simulink model "Wireless_Charging_Old_V1"  (R2022b)
settings: Solver=VariableStepAuto  StartTime=0.0  StopTime=5  RelTol=1e-3
libraries: spsVoltageMeasurementLib x16, spsSeriesRLCBranchLib x12, spsDiodeLib x11, spsIGBTDiodeLib x9, spsCurrentMeasurementLib x7, spsMosfetLib x2, spsACVoltageSourceLib x1, spsPWMGeneratorDCDCLib x1, spsPWMGenerator2LevelLib x1, spsGroundLib x1, spsMutualInductanceLib x1, spspowerguiLib x1
settings Model: Creator=hp  LastModifiedBy=Aryan Aggarwal
settings OptimizationCC: ReuseModelBlockBuffer=on

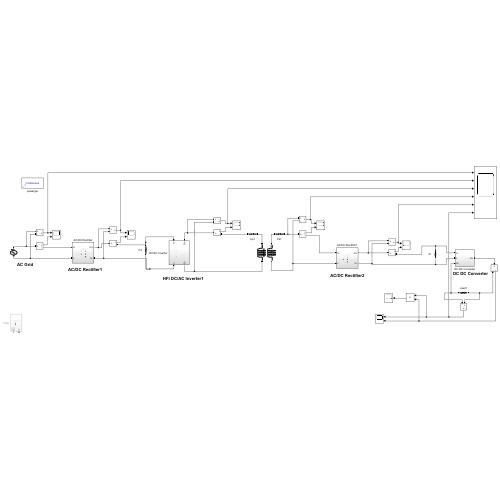
[thumbnail: Simulink's stored preview of the top-level diagram]
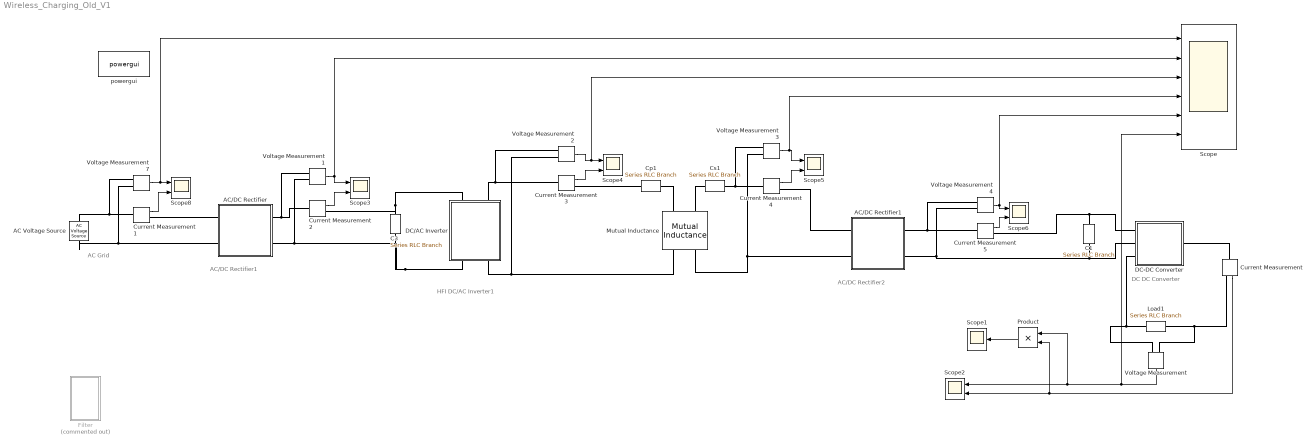
== system Wireless_Charging_Old_V1 ==
  note: AC/DC Rectifier1
  note: AC Grid
  note: HFI DC/AC Inverter1
  note: AC/DC Rectifier2
  note: DC DC Converter
  AC Voltage Source : spsACVoltageSourceLib/AC Voltage Source  Amplitude=230  Phase=0  Frequency=50  SampleTime=0  Measurements=None  BusType=swing  Pref=10e3  Qref=0  Qmin=-inf  Qmax=+inf
  AC/DC Rectifier : Subsystem
  AC/DC Rectifier1 : Subsystem
  C1 : spsSeriesRLCBranchLib/Series RLC Branch  LConnTagsString=__new0  RConnTagsString=__new0  BranchType=C  Resistance=1  Inductance=1e-3  SetiL0=off  InitialCurrent=0  Capacitance=1  Setx0=off  InitialVoltage=0  Measurements=None
  C3 : spsSeriesRLCBranchLib/Series RLC Branch  LConnTagsString=__new0  RConnTagsString=__new0  BranchType=C  Resistance=1  Inductance=1e-3  SetiL0=off  InitialCurrent=0  Capacitance=1  Setx0=off  InitialVoltage=0  Measurements=None
  Cp1 : spsSeriesRLCBranchLib/Series RLC Branch  LConnTagsString=__new0  RConnTagsString=__new0  BranchType=C  Resistance=1  Inductance=1e-3  SetiL0=off  InitialCurrent=0  Capacitance=4.67e-03  Setx0=off  InitialVoltage=0  Measurements=None
  Cs1 : spsSeriesRLCBranchLib/Series RLC Branch  LConnTagsString=__new0  RConnTagsString=__new0  BranchType=C  Resistance=1  Inductance=1e-3  SetiL0=off  InitialCurrent=0  Capacitance=4.67e-03  Setx0=off  InitialVoltage=0  Measurements=None
  Current Measurement{,1..5} (6 alike) : spsCurrentMeasurementLib/Current Measurement  PhasorSimulation=off  OutputType=Complex  PSBequivalent=0
  DC-DC Converter : Subsystem
  DC/AC Inverter : Subsystem
  Filter : Subsystem  Commented=on
  Load1 : spsSeriesRLCBranchLib/Series RLC Branch  LConnTagsString=__new0  RConnTagsString=__new0  BranchType=R  Resistance=100  Inductance=1e-3  SetiL0=off  InitialCurrent=0  Capacitance=1000e-6  Setx0=off  InitialVoltage=0  Measurements=None
  Mutual Inductance : spsMutualInductanceLib/Mutual Inductance  LConnTagsString=a|b  RConnTagsString=A|B  TypeOfMutual=Two or three windings with equal mutual terms  NumberOfWindings=3  SelfImpedance1=[1.1 30e-03]  SelfImpedance2=[ 1.1 30e-03]  ThreeWindings=off  SelfImpedance3=[ 1.1 1.1e-03]  MutualImpedance=[1.0 29e-03]  InductanceMatrix="[1.0 0.9  0.9 ;  0.9 1.0  0.9;  0.9 0.9 1.0 ] * 1e-3"  ResistanceMatrix="[1.0 0.9  0.9 ;  0.9 1.0  0.9;  0.9 0.9 1.0 ]"  Measurements=None
      settings: LibrarySourceBlock=sps_lib/Passives/Mutual Inductance
  Product : Product
  Scope : Scope  NumInputPorts=6
  Scope1 : Scope
  Scope{2..6,8} (6 alike) : Scope  NumInputPorts=2
  Voltage Measurement{,1..4,7} (6 alike) : spsVoltageMeasurementLib/Voltage Measurement  PhasorSimulation=off  OutputType=Complex  PSBequivalent=0
  powergui : spspowerguiLib/powergui  Priority=1  SimulationMode=Continuous  SampleTime=50e-6  frequency=60  Iterations=50  frequencyindice=0  Pbase=100e6  ErrMax=1e-4  UnitsV=kV  UnitsW=MW  buscounter=0  FunctionMessages=off  echomessages=off  EnableUseOfTLC=off  CurrentSourceSwitches=off  DisableSnubberDevices=off  DisableRonSwitches=off  DisableVfSwitches=off  DisplayEquations=off  AutomaticDiscreteSolvers=off  SolverType=Tustin/Backward Euler (TBE)  Interpol=off  ExternalGateDelay=off  methode=off  Ts=100  x0status=blocks  SPID=on  SwTol=0  HookPort=off  NonlinearTolerance=1e-4  nMaxIteration=100  ContinueOnMaxIteration=off  RestoreLinks=warning  ResistiveCurrentMeasurement=off  Frange=[0:2:500]  Ylog=off  Xlog=on  ShowGrid=off  save=off  variable=ZData  structure=0  ZoomFFT=off  StartTime=0.0  cycles=1  DisplayStyle=1  fundamental=60  FreqAxis=off  MaxFrequency=1000  frequencyindicesteady=1  RmsSteady=1  display=off
  wires:
  Product/1 -> Scope1/1
  Voltage Measurement7/1 -> Scope/1, Scope8/1
  Current Measurement1/1 -> Scope8/2
  Voltage Measurement1/1 -> Scope3/1, Scope/2
  Current Measurement2/1 -> Scope3/2
  Voltage Measurement2/1 -> Scope/3, Scope4/1
  Current Measurement3/1 -> Scope4/2
  Voltage Measurement3/1 -> Scope/4, Scope5/1
  Current Measurement4/1 -> Scope5/2
  Voltage Measurement4/1 -> Scope6/1, Scope/5
  Current Measurement5/1 -> Scope6/2
  Voltage Measurement/1 -> Scope2/1, Product/1, Scope/6
  Current Measurement/1 -> Scope2/2, Product/2
  connections:
  Current Measurement/LConn1 -- DC-DC Converter/RConn1
  C1/RConn1 -- DC-DC Converter/LConn2 -- Voltage Measurement4/LConn2 -- AC/DC Rectifier1/LConn2
  Voltage Measurement3/LConn2 -- Mutual Inductance/RConn2 -- AC/DC Rectifier1/RConn2
  DC-DC Converter/LConn3 -- Load1/RConn1 -- Voltage Measurement/LConn2
  Current Measurement5/RConn1 -- C1/LConn1 -- DC-DC Converter/LConn1
  DC/AC Inverter/RConn2 -- Voltage Measurement2/LConn2 -- Mutual Inductance/RConn1
  Voltage Measurement/LConn1 -- Load1/LConn1 -- Current Measurement/RConn1
  Cp1/RConn1 -- Mutual Inductance/LConn1
  AC Voltage Source/LConn1 -- Voltage Measurement7/LConn2 -- AC/DC Rectifier/RConn2
  Cs1/LConn1 -- Mutual Inductance/LConn2
  Current Measurement1/RConn1 -- AC/DC Rectifier/RConn1
  Current Measurement1/LConn1 -- Voltage Measurement7/LConn1 -- AC Voltage Source/RConn1
  C3/LConn1 -- Current Measurement2/RConn1 -- DC/AC Inverter/LConn1
  C3/RConn1 -- Voltage Measurement1/LConn2 -- AC/DC Rectifier/LConn2 -- DC/AC Inverter/RConn1
  Current Measurement2/LConn1 -- Voltage Measurement1/LConn1 -- AC/DC Rectifier/LConn1
  Current Measurement3/LConn1 -- Voltage Measurement2/LConn1 -- DC/AC Inverter/LConn2
  Current Measurement3/RConn1 -- Cp1/LConn1
  Current Measurement4/LConn1 -- Voltage Measurement3/LConn1 -- Cs1/RConn1
  Current Measurement4/RConn1 -- AC/DC Rectifier1/RConn1
  Current Measurement5/LConn1 -- Voltage Measurement4/LConn1 -- AC/DC Rectifier1/LConn1

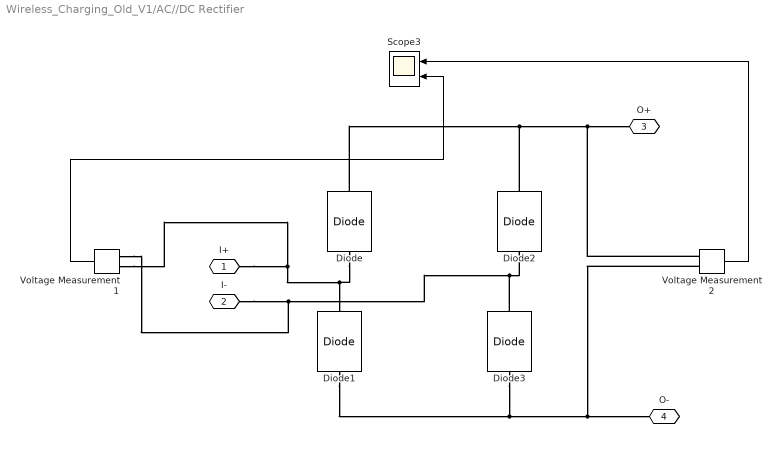
== system Wireless_Charging_Old_V1/AC//DC Rectifier ==
  Diode{,1..3} (4 alike) : spsDiodeLib/Diode  Ron=0.001  Lon=0  Vf=0.8  IC=0  UseSnubber=0  Rs=500  Cs=250e-9  Measurements=off
  Scope3 : Scope  NumInputPorts=2
  Voltage Measurement1 : spsVoltageMeasurementLib/Voltage Measurement  PhasorSimulation=off  OutputType=Complex  PSBequivalent=0
  Voltage Measurement2 : spsVoltageMeasurementLib/Voltage Measurement  PhasorSimulation=off  OutputType=Complex  PSBequivalent=0
  I+ : PMIOPort  Side=Right
  I- : PMIOPort  Port=2  Side=Right
  O+ : PMIOPort  Port=3  Side=Left
  O- : PMIOPort  Port=4  Side=Left
  wires:
  Voltage Measurement2/1 -> Scope3/1
  Voltage Measurement1/1 -> Scope3/2
  connections:
  Diode3/RConn1 -- Voltage Measurement1/LConn2 -- I-/RConn1 -- Diode2/LConn1
  Diode/LConn1 -- Voltage Measurement1/LConn1 -- I+/RConn1 -- Diode1/RConn1
  Diode/RConn1 -- Voltage Measurement2/LConn1 -- O+/RConn1 -- Diode2/RConn1
  Diode1/LConn1 -- Diode3/LConn1 -- Voltage Measurement2/LConn2 -- O-/RConn1

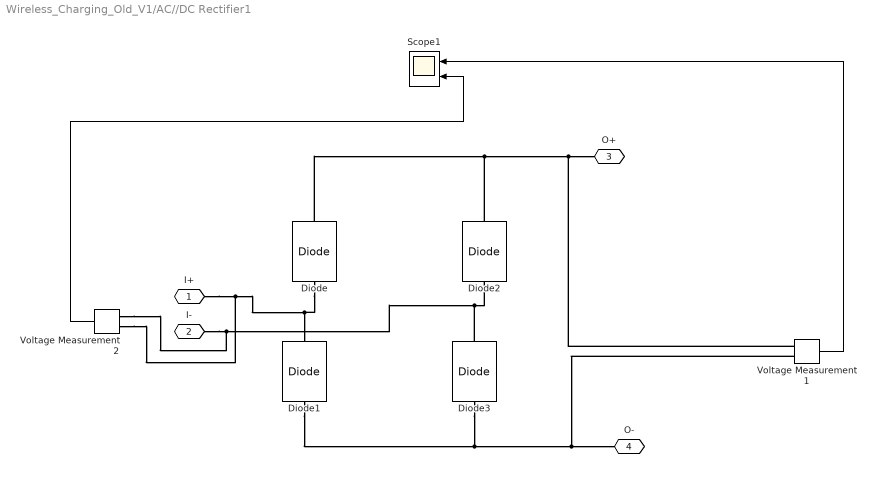
== system Wireless_Charging_Old_V1/AC//DC Rectifier1 ==
  Diode{,1..3} (4 alike) : spsDiodeLib/Diode  Ron=0.001  Lon=0  Vf=0.8  IC=0  UseSnubber=0  Rs=500  Cs=250e-9  Measurements=off
  Scope1 : Scope  NumInputPorts=2
  Voltage Measurement1 : spsVoltageMeasurementLib/Voltage Measurement  PhasorSimulation=off  OutputType=Complex  PSBequivalent=0
  Voltage Measurement2 : spsVoltageMeasurementLib/Voltage Measurement  PhasorSimulation=off  OutputType=Complex  PSBequivalent=0
  I+ : PMIOPort  Side=Right
  I- : PMIOPort  Port=2  Side=Right
  O+ : PMIOPort  Port=3  Side=Left
  O- : PMIOPort  Port=4  Side=Left
  wires:
  Voltage Measurement1/1 -> Scope1/1
  Voltage Measurement2/1 -> Scope1/2
  connections:
  Diode3/RConn1 -- Voltage Measurement2/LConn2 -- I-/RConn1 -- Diode2/LConn1
  Diode/LConn1 -- Voltage Measurement2/LConn1 -- I+/RConn1 -- Diode1/RConn1
  Diode/RConn1 -- Diode2/RConn1 -- Voltage Measurement1/LConn1 -- O+/RConn1
  Diode1/LConn1 -- Diode3/LConn1 -- Voltage Measurement1/LConn2 -- O-/RConn1

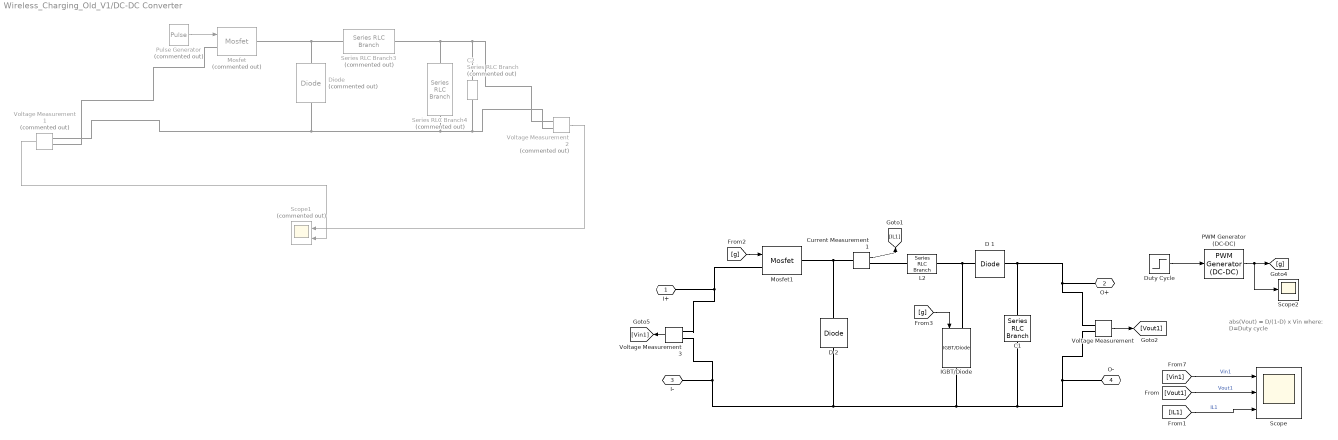
== system Wireless_Charging_Old_V1/DC-DC Converter ==
  note: abs(Vout) = D/(1-D) x Vin
      | where: D=Duty cycle
  C1 : spsSeriesRLCBranchLib/Series RLC Branch  LConnTagsString=__new0  RConnTagsString=__new0  BranchType=C  Resistance=1e-4  Inductance=200e-6  SetiL0=off  InitialCurrent=0  Capacitance=2000e-6  Setx0=on  InitialVoltage=7.5  Measurements=None
  C2 : spsSeriesRLCBranchLib/Series RLC Branch  Commented=on  LConnTagsString=__new0  RConnTagsString=__new0  BranchType=C  Resistance=1  Inductance=1e-3  SetiL0=off  InitialCurrent=0  Capacitance=1  Setx0=off  InitialVoltage=0  Measurements=None
  Current Measurement1 : spsCurrentMeasurementLib/Current Measurement  PhasorSimulation=off  OutputType=Complex  PSBequivalent=0
  D 1 : spsDiodeLib/Diode  Ron=1e-3  Lon=0  Vf=0  IC=0  UseSnubber=off  Rs=inf  Cs=inf  Measurements=off
  D 2 : spsDiodeLib/Diode  Ron=1e-3  Lon=0  Vf=0  IC=0  UseSnubber=off  Rs=inf  Cs=inf  Measurements=off
  Diode : spsDiodeLib/Diode  Commented=on  Ron=0.001  Lon=0  Vf=0.8  IC=0  UseSnubber=0  Rs=500  Cs=250e-9  Measurements=off
  Duty Cycle : Step  Time=0.015  Before=0.456  After=0.602  SampleTime=0
  IGBT/Diode : spsIGBTDiodeLib/IGBT//Diode  Ron=1e-3  Rs=1e5  Cs=inf  Measurements=off
  L2 : spsSeriesRLCBranchLib/Series RLC Branch  LConnTagsString=__new0  RConnTagsString=__new0  BranchType=L  Resistance=1e-4  Inductance=750e-6  SetiL0=on  InitialCurrent=14  Capacitance=30e-6  Setx0=off  InitialVoltage=150  Measurements=None
  Mosfet : spsMosfetLib/Mosfet  Commented=on  Ron=0.1  Lon=0  Rd=0.01  Vfd=0  IC=0  Rs=1e5  Cs=inf  Measurements=off
  Mosfet1 : spsMosfetLib/Mosfet  Ron=1e-3  Lon=0  Rd=1e-3  Vfd=0  IC=0  Rs=1e6  Cs=inf  Measurements=off
  PWM Generator (DC-DC) : spsPWMGeneratorDCDCLib/PWM Generator (DC-DC)  Fsw=10e3  Ts=0
  Pulse Generator : DiscretePulseGenerator  Commented=on  PulseType=Time based  Period=1/100  PulseWidth=80
  Scope : Scope  NumInputPorts=3
  Scope1 : Scope  Commented=on  NumInputPorts=2
  Scope2 : Scope
  Series RLC Branch3 : spsSeriesRLCBranchLib/Series RLC Branch  Commented=on  LConnTagsString=__new0  RConnTagsString=__new0  BranchType=L  Resistance=1  Inductance=50e-3  SetiL0=off  InitialCurrent=0  Capacitance=1e-6  Setx0=off  InitialVoltage=0  Measurements=None
  Series RLC Branch4 : spsSeriesRLCBranchLib/Series RLC Branch  Commented=on  LConnTagsString=__new0  RConnTagsString=__new0  BranchType=C  Resistance=1  Inductance=1e-3  SetiL0=off  InitialCurrent=0  Capacitance=100e-6  Setx0=off  InitialVoltage=0  Measurements=None
  Voltage Measurement : spsVoltageMeasurementLib/Voltage Measurement  PhasorSimulation=off  OutputType=Complex  PSBequivalent=0
  Voltage Measurement1 : spsVoltageMeasurementLib/Voltage Measurement  Commented=on  PhasorSimulation=off  OutputType=Complex  PSBequivalent=0
  Voltage Measurement2 : spsVoltageMeasurementLib/Voltage Measurement  Commented=on  PhasorSimulation=off  OutputType=Complex  PSBequivalent=0
  Voltage Measurement3 : spsVoltageMeasurementLib/Voltage Measurement  PhasorSimulation=off  OutputType=Complex  PSBequivalent=0
  I+ : PMIOPort  Side=Left
  O+ : PMIOPort  Port=2  Side=Right
  I- : PMIOPort  Port=3  Side=Left
  O- : PMIOPort  Port=4  Side=Left
  wires:
  Pulse Generator/1 -> Mosfet/1
  Voltage Measurement1/1 -> Scope1/2
  Voltage Measurement2/1 -> Scope1/1
  Current Measurement1/1 -> [IL1]
  [g] -> IGBT/Diode/1
  Voltage Measurement/1 -> [Vout1]
  [g] -> Mosfet1/1
  Voltage Measurement3/1 -> [Vin1]
  Duty Cycle/1 -> PWM Generator (DC-DC)/1
  PWM Generator (DC-DC)/1 -> Scope2/1, [g]
  [IL1] -> Scope/3  "IL1"
  [Vout1] -> Scope/2  "Vout1"
  [Vin1] -> Scope/1  "Vin1"
  connections:
  Series RLC Branch3/LConn1 -- Mosfet/RConn1 -- Diode/RConn1
  Series RLC Branch4/LConn1 -- Series RLC Branch3/RConn1 -- C2/RConn1 -- Voltage Measurement2/LConn1
  Voltage Measurement2/LConn2 -- Series RLC Branch4/RConn1 -- Voltage Measurement1/LConn2 -- Diode/LConn1 -- C2/LConn1
  Voltage Measurement1/LConn1 -- Mosfet/LConn1
  IGBT/Diode/LConn1 -- D 1/LConn1 -- L2/RConn1
  Voltage Measurement/LConn2 -- C1/RConn1 -- IGBT/Diode/RConn1 -- D 2/LConn1 -- Voltage Measurement3/LConn2 -- I-/RConn1 -- O-/RConn1
  Voltage Measurement/LConn1 -- C1/LConn1 -- D 1/RConn1 -- O+/RConn1
  I+/RConn1 -- Mosfet1/LConn1 -- Voltage Measurement3/LConn1
  Current Measurement1/LConn1 -- Mosfet1/RConn1 -- D 2/RConn1
  L2/LConn1 -- Current Measurement1/RConn1

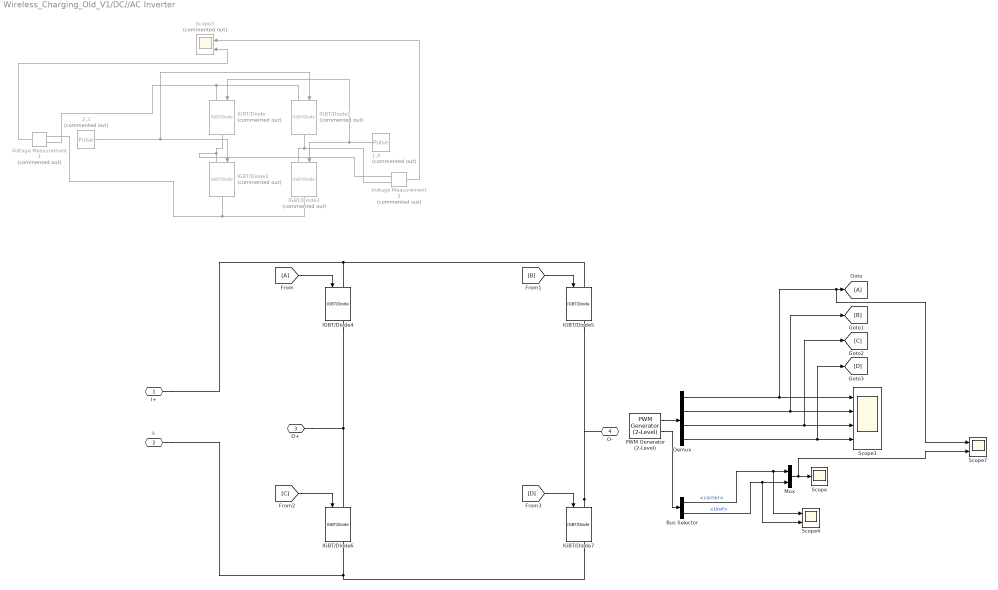
== system Wireless_Charging_Old_V1/DC//AC Inverter ==
  1,4 : DiscretePulseGenerator  Commented=on  PulseType=Time based  Amplitude=15  Period=1/50  PulseWidth=50  PhaseDelay=1/100
  2,3 : DiscretePulseGenerator  Commented=on  PulseType=Time based  Amplitude=15  Period=1/50  PulseWidth=50
  Bus Selector : BusSelector  OutputSignals=carrier,Uref
  Demux : Demux
  From : From
  Goto : Goto
  IGBT/Diode{,1..3} (4 alike) : spsIGBTDiodeLib/IGBT//Diode  Commented=on  Ron=1e-3  Rs=1e5  Cs=inf  Measurements=off
  IGBT/Diode{4..7} (4 alike) : spsIGBTDiodeLib/IGBT//Diode  Ron=1e-3  Rs=1e5  Cs=inf  Measurements=on
  Mux : Mux  Inputs=2
  PWM Generator (2-Level) : spsPWMGenerator2LevelLib/PWM Generator (2-Level)  ModulatorType=Single-phase full-bridge - Bipolar modulation (4 pulses)  ModulatorMode=Unsynchronized  Fc=20000  Pc=0  nF=27  MinMax="[ -1  1 ]"  SamplingTechnique=Asymmetrical regular (double edge)  ModulatingSignals=on  m=0.75  Freq=60  Phase=0  Ts=0  ShowCarrierOutport=on
  Scope : Scope
  Scope1 : Scope  NumInputPorts=4
  Scope3 : Scope  Commented=on  NumInputPorts=2
  Scope4 : Scope  NumInputPorts=2
  Scope7 : Scope  NumInputPorts=2
  Voltage Measurement1 : spsVoltageMeasurementLib/Voltage Measurement  Commented=on  PhasorSimulation=off  OutputType=Complex  PSBequivalent=0
  Voltage Measurement2 : spsVoltageMeasurementLib/Voltage Measurement  Commented=on  PhasorSimulation=off  OutputType=Complex  PSBequivalent=0
  I+ : PMIOPort  Side=Left
  I- : PMIOPort  Port=2  Side=Right
  O+ : PMIOPort  Port=3  Side=Left
  O- : PMIOPort  Port=4  Side=Right
  wires:
  2,3/1 -> IGBT/Diode1/1, IGBT/Diode2/1
  1,4/1 -> IGBT/Diode3/1, IGBT/Diode/1
  Voltage Measurement2/1 -> Scope3/1
  Voltage Measurement1/1 -> Scope3/2
  From/1 -> IGBT/Diode4/1
  Bus Selector/2 -> Scope4/2, Mux/2  "<Uref>"
  Demux/2 -> [B], Scope1/2
  Bus Selector/1 -> Scope4/1, Mux/1  "<carrier>"
  PWM Generator (2-Level)/1 -> Demux/1
  [C] -> IGBT/Diode6/1
  [B] -> IGBT/Diode5/1
  Demux/1 -> Scope7/1, Goto/1, Scope1/1
  [D] -> IGBT/Diode7/1
  Demux/4 -> [D], Scope1/4
  Demux/3 -> [C], Scope1/3
  Mux/1 -> Scope7/2, Scope/1
  PWM Generator (2-Level)/2 -> Bus Selector/1
  connections:
  IGBT/Diode1/LConn1 -- Voltage Measurement1/LConn1 -- IGBT/Diode/LConn1
  IGBT/Diode3/RConn1 -- Voltage Measurement1/LConn2 -- IGBT/Diode2/RConn1
  Voltage Measurement2/LConn1 -- IGBT/Diode/RConn1 -- IGBT/Diode2/LConn1
  Voltage Measurement2/LConn2 -- IGBT/Diode3/LConn1 -- IGBT/Diode1/RConn1
  IGBT/Diode6/LConn1 -- O+/RConn1 -- IGBT/Diode4/RConn1
  IGBT/Diode7/LConn1 -- O-/RConn1 -- IGBT/Diode5/RConn1
  IGBT/Diode6/RConn1 -- IGBT/Diode7/RConn1 -- I-/RConn1
  IGBT/Diode4/LConn1 -- I+/RConn1 -- IGBT/Diode5/LConn1

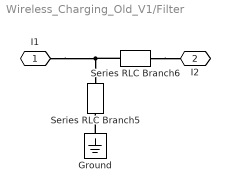
== system Wireless_Charging_Old_V1/Filter ==
  Ground : spsGroundLib/Ground  LConnTagsString=a
  Series RLC Branch5 : spsSeriesRLCBranchLib/Series RLC Branch  LConnTagsString=__new0  RConnTagsString=__new0  BranchType=C  Resistance=1  Inductance=1e-3  SetiL0=off  InitialCurrent=0  Capacitance=100e-6  Setx0=off  InitialVoltage=0  Measurements=None
  Series RLC Branch6 : spsSeriesRLCBranchLib/Series RLC Branch  LConnTagsString=__new0  RConnTagsString=__new0  BranchType=L  Resistance=1  Inductance=470e-2  SetiL0=off  InitialCurrent=0  Capacitance=4.961e-03  Setx0=off  InitialVoltage=0  Measurements=None
  I1 : PMIOPort  Side=Right
  I2 : PMIOPort  Port=2  Side=Right
  connections:
  Ground/LConn1 -- Series RLC Branch5/LConn1
  Series RLC Branch6/RConn1 -- I2/RConn1
  Series RLC Branch6/LConn1 -- I1/RConn1 -- Series RLC Branch5/RConn1
